simulink model "Assignment1Problem1"  (R2017b)
settings: Solver=VariableStepAuto  StartTime=0.0  StopTime=10.0  RelTol=1e-3
libraries: simulink_extras x1
settings Model: Creator=alexbenasutti  LastModifiedBy=alexbenasutti

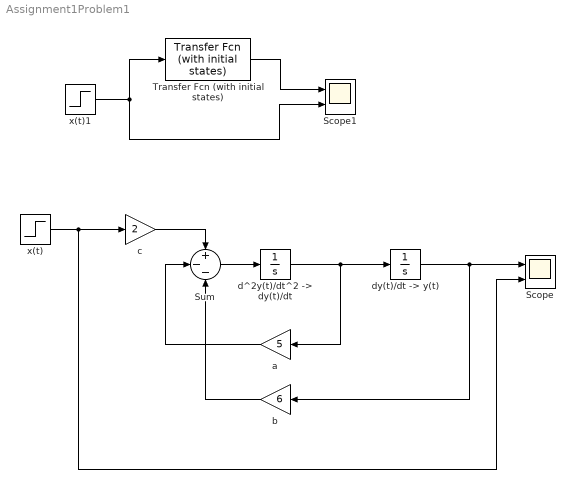
== system Assignment1Problem1 ==
  Scope : Scope  NumInputPorts=2
  Scope1 : Scope  NumInputPorts=2
  Sum : Sum  Inputs=+--
  Transfer Fcn (with initial states) : simulink_extras/Additional Linear/Transfer Fcn (with initial states)  N=[2]  D=[1 5 6]  X0=0 -1
  "a " : Gain  Gain=5
  b : Gain  Gain=6
  "c " : Gain  Gain=2
  "d^2y(t)/dt^2 -> dy(t)/dt" : Integrator
  "dy(t)/dt -> y(t)" : Integrator  InitialCondition=-1
  x(t) : Step  SampleTime=0
  x(t)1 : Step  SampleTime=0
  wires:
  Sum/1 -> "d^2y(t)/dt^2 -> dy(t)/dt"/1
  "a "/1 -> Sum/2
  b/1 -> Sum/3
  "c "/1 -> Sum/1
  x(t)/1 -> Scope/2, "c "/1
  "d^2y(t)/dt^2 -> dy(t)/dt"/1 -> "a "/1, "dy(t)/dt -> y(t)"/1
  "dy(t)/dt -> y(t)"/1 -> b/1, Scope/1
  Transfer Fcn (with initial states)/1 -> Scope1/1
  x(t)1/1 -> Scope1/2, Transfer Fcn (with initial states)/1
